simulink model "CBuilderDemo"  (R2014a)
settings: Solver=ode45  StartTime=0.0  StopTime=10.0  RelTol=1e-3
settings Model: Creator=李广文  LastModifiedBy=李广文

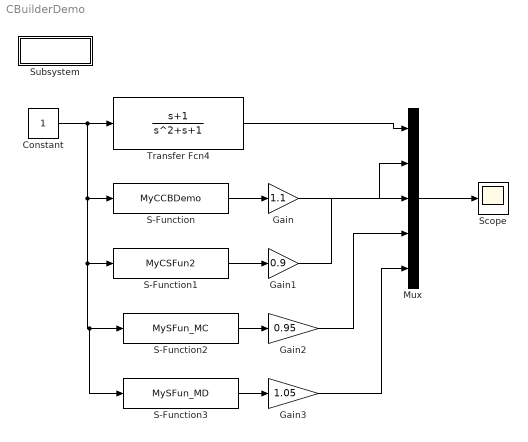
== system CBuilderDemo ==
  Constant : Constant
  Gain : Gain  Gain=1.1
  Gain1 : Gain  Gain=0.9
  Gain2 : Gain  Gain=0.95
  Gain3 : Gain  Gain=1.05
  Mux : Mux  Inputs=5
  S-Function : S-Function  FunctionName=MyCCBDemo  EnableBusSupport=off
  S-Function1 : S-Function  FunctionName=MyCSFun2  EnableBusSupport=off
  S-Function2 : S-Function  FunctionName=MySFun_MC  EnableBusSupport=off
  S-Function3 : S-Function  FunctionName=MySFun_MD  EnableBusSupport=off
  Scope : Scope
  Subsystem : Subsystem
      settings: OpenFcn=|
      | clc
      | G=tf([1,1],[1,1,1])
      | [A,B,C,D]=ssdata(G);
  Transfer Fcn4 : TransferFcn  Numerator=[1 1]  Denominator=[1 1 1]
  wires:
  Constant/1 -> S-Function3/1, S-Function2/1, S-Function1/1, S-Function/1, Transfer Fcn4/1
  Transfer Fcn4/1 -> Mux/1
  Mux/1 -> Scope/1
  S-Function/1 -> Gain/1
  S-Function1/1 -> Gain1/1
  Gain/1 -> Mux/2
  Gain1/1 -> Mux/3
  S-Function2/1 -> Gain2/1
  Gain2/1 -> Mux/4
  S-Function3/1 -> Gain3/1
  Gain3/1 -> Mux/5

== system CBuilderDemo/Subsystem ==
